simulink model "Group3_HEV_model"  (Simulink 7.9)
settings: Solver=ode4  StartTime=0.0  StopTime=Stoptime  FixedStep=1  MaxStep=.05  RelTol=1e-3
InitFcn:
  | load Mat_files/ENV_Data.mat;
  | load Mat_files/TRAN_Data.mat;
  | load Mat_files/VEH_Data.mat;
  | load Mat_files/TC_Data.mat;
  | load Mat_files/Drive_cycle.mat;
  | load Mat_files/ICE_Data.mat;
  | load Mat_files/EM_Data.mat;
  | load Mat_files/BATT_Data.mat
  | clc;
  | %warning off all;
StopFcn:
  | disp('Simulation Complete.')
values from neighbouring files (symbols this model uses):
  EM = EM2    [Group3_Plot.m]
  EM2 =     [EM2_map.mat]
  em_trq_e_g1 = em_trq_e    [Group3_ECMS_control_strategy.m]    (also in ecms_table_n5.mat = [-2 -2 -2 -2 -2 -2 -2 -2 -2 -2 -2 -2 ... (715 elements, 11x1)
  em_trq_e_g2 = em_trq_e    [Group3_ECMS_control_strategy.m]    (also in ecms_table_n5.mat = [-2 -2 -2 -2 -2 -2 -2 -2 -2 -2 -2 -2 ... (715 elements, 11x1)
  em_trq_e_g3 = em_trq_e    [Group3_ECMS_control_strategy.m]    (also in ecms_table_n5.mat = [-2 -2 -2 -2 -2 -2 -2 -2 -2 -2 -2 -2 ... (715 elements, 11x1)
  fs_0 = 1    [Group3_Initialization.m]
  fs_act = 1    [Group3_Initialization.m]
  hA_0 = 0.07    [Group3_Initialization.m]
  ICE =     [Engine2_map.mat]
  ice_w_e = linspace(0,50*m2,m2+1)    [Group3_ECMS_control_strategy.m]    (also in ecms_table_n5.mat = [0 50 100 150 200 250 300 350 400 450 500])
  mc = 50    [Group3_Initialization.m]
  N = 250    [Group3_Initialization.m]
  soc_e = linspace(-1,1,m3)    [Group3_ECMS_control_strategy.m]    (also in ecms_table_n5.mat = [-1 -0.5 0 0.5 1])
  soc_h = 0.85    [Group3_ECMS_control_strategy.m]    (also in Group3_Initialization.m)
  soc_l = 0.55    [Group3_ECMS_control_strategy.m]    (also in Group3_Initialization.m)
  Sport = 1    [Group3_Initialization.m]
  T_amb = 20+273    (= 293)    [Group3_Initialization.m]
  Treq = linspace(0,20*m1,m1+1)    [Group3_ECMS_control_strategy.m]    (also in ecms_table_n5.mat = [0 20 40 60 80 100 120 140 160 180 200 220 ... (13 elements,)
undefined symbols (not defined in the file or in its folder): BATT, ENV, TC, TRAN, VEH
libraries: simulink x6
(part 1 of 2)
settings Model: Creator=pisup  LastModifiedBy=HarryBrown
settings OptimizationCC: InitFltsAndDblsToZero=on
settings DebuggingCC: SaveWithParameterizedLinksMsg=none  CheckSSInitialOutputMsg=off  SignalResolutionControl=TryResolveAllWithWarning  MultiTaskDSMMsg=warning  MultiTaskCondExecSysMsg=none  StrictBusMsg=None
settings RTWCC: IncludeERTFirstTime=on
settings CodeAppCC: CustomSymbolStrType=$N$R$M_T
settings GRTTargetCC: TargetFcnLib=ansi_tfl_tmw.mat  CombineOutputUpdateFcns=off  GRTInterface=on

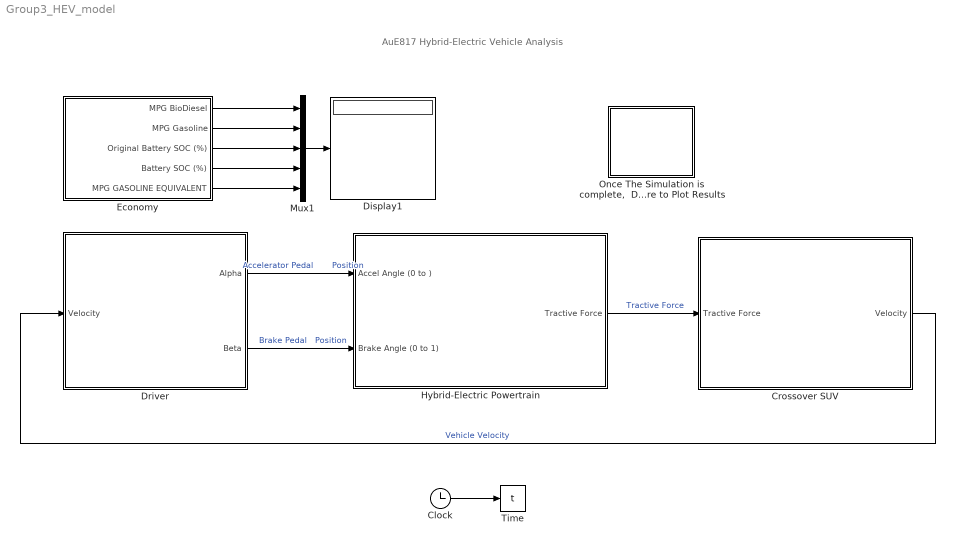
== system Group3_HEV_model ==
  note: AuE817
      | Hybrid-Electric Vehicle Analysis
  Clock : Clock
  Crossover SUV : Subsystem
      mask Type: Vehicle
      mask Display: image(imread('Images\Equinox.jpg'))
  Display1 : Display
  Driver : Subsystem
      mask Display: image(imread('Images\Driver.jpg'))
  Economy : Subsystem
      mask Type: Fuel Economy
  Hybrid-Electric Powertrain : Subsystem
      mask Display: image(imread('Images\PT.jpg'))
  Mux1 : Mux  Inputs=5
  "Once The Simulation is complete,  Double Click Here to Plot Results" : Subsystem
      settings: OpenFcn=eval 'Plot_Results'
  Time : ToWorkspace  VariableName=t  SampleTime=-1
  wires:
  Crossover SUV/1(Velocity) -> Driver/1(" Velocity")  "Vehicle Velocity"
  Driver/2(Beta) -> Hybrid-Electric Powertrain/2("Brake Angle (0 to 1) ")  "Brake Pedal   Position"
  Driver/1(Alpha) -> Hybrid-Electric Powertrain/1("Accel Angle (0 to ) ")  "Accelerator Pedal       Position"
  Hybrid-Electric Powertrain/1(Tractive Force) -> Crossover SUV/1(Tractive Force)  "Tractive Force"
  Clock/1 -> Time/1
  Mux1/1 -> Display1/1
  Economy/1(MPG BioDiesel) -> Mux1/1
  Economy/2(MPG Gasoline) -> Mux1/2
  Economy/3(Original Battery SOC (%)) -> Mux1/3
  Economy/5(MPG GASOLINE EQUIVALENT) -> Mux1/5
  Economy/4(Battery SOC (%)) -> Mux1/4

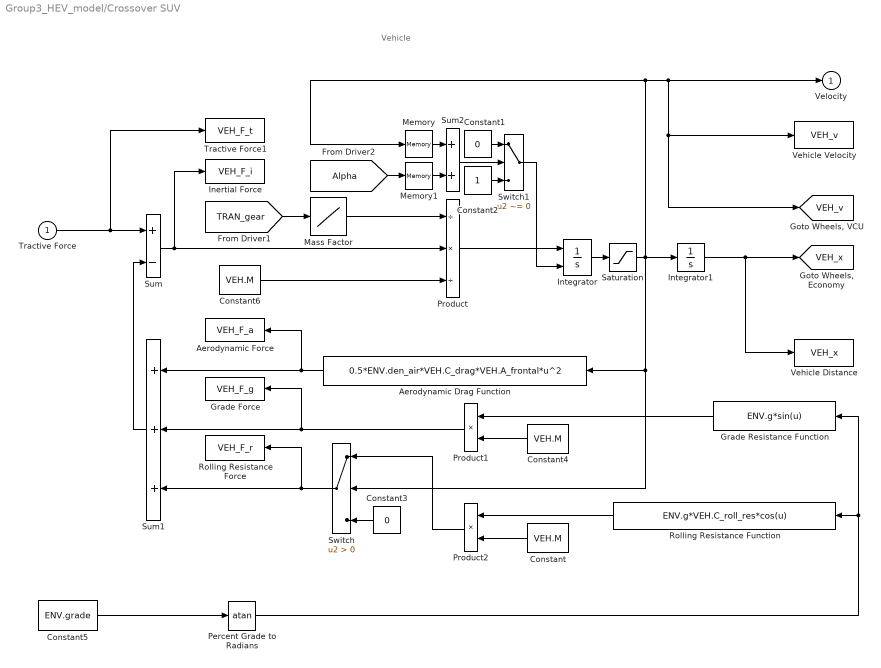
== system Group3_HEV_model/Crossover SUV ==
  note: Vehicle
  Tractive Force : Inport
  Aerodynamic Drag Function : Fcn  Expr=0.5*ENV.den_air*VEH.C_drag*VEH.A_frontal*u^2
  Aerodynamic Force : ToWorkspace  VariableName=VEH_F_a  SampleTime=-1
  Constant : Constant  Value=VEH.M
  Constant1 : Constant  Value=0
  Constant2 : Constant
  Constant3 : Constant  Value=0
  Constant4 : Constant  Value=VEH.M
  Constant5 : Constant  Value=ENV.grade
  Constant6 : Constant  Value=VEH.M
  Grade Force : ToWorkspace  VariableName=VEH_F_g  SampleTime=-1
  Grade Resistance Function : Fcn  Expr=ENV.g*sin(u)
  Inertial Force : ToWorkspace  VariableName=VEH_F_i  SampleTime=-1
  Integrator : Integrator  ExternalReset=level  LowerSaturationLimit=0
  Integrator1 : Integrator
  Mass Factor : Lookup  InputValues=[1 2 3 4 5 6]  Table=[1.7896 1.3703 1.2188 1.1536 1.1093 1.085]  SaturateOnIntegerOverflow=on
  Memory : Memory
  Memory1 : Memory
  Percent Grade to Radians : Trigonometry  Operator=atan
  Product : Product  Inputs=/*/  RndMeth=Zero
  Product1 : Product  Inputs=**  RndMeth=Zero
  Product2 : Product  Inputs=**  RndMeth=Zero
  Rolling Resistance Force : ToWorkspace  VariableName=VEH_F_r  SampleTime=-1
  Rolling Resistance Function : Fcn  Expr=ENV.g*VEH.C_roll_res*cos(u)
  Saturation : Saturate  UpperLimit=inf  LowerLimit=0
  Sum : Sum  Inputs=+-  SaturateOnIntegerOverflow=on  InputSameDT=on  OutDataTypeStr=Inherit: Same as first input
  Sum1 : Sum  Inputs=+++  SaturateOnIntegerOverflow=on  InputSameDT=on  OutDataTypeStr=Inherit: Same as first input
  Sum2 : Sum  SaturateOnIntegerOverflow=on  InputSameDT=on  OutDataTypeStr=Inherit: Same as first input
  Switch : Switch  Criteria=u2 > Threshold  SaturateOnIntegerOverflow=on  InputSameDT=on
  Switch1 : Switch  Criteria=u2 ~= 0  SaturateOnIntegerOverflow=on  InputSameDT=on
  Tractive Force1 : ToWorkspace  VariableName=VEH_F_t  SampleTime=-1
  Vehicle Distance : ToWorkspace  VariableName=VEH_x  SampleTime=-1
  Vehicle Velocity : ToWorkspace  VariableName=VEH_v  SampleTime=-1
  Velocity : Outport  InitialOutput=0
  tag scope: VEH_v=global, VEH_x=global
  wires:
  Sum1/1 -> Sum/2
  Tractive Force/1 -> Sum/1, Tractive Force1/1
  Aerodynamic Drag Function/1 -> Aerodynamic Force/1, Sum1/1
  Integrator1/1 -> [VEH_x], Vehicle Distance/1
  Constant3/1 -> Switch/3
  Sum/1 -> Inertial Force/1, Product/2
  Integrator/1 -> Saturation/1
  Switch/1 -> Sum1/3, Rolling Resistance Force/1
  Constant5/1 -> Percent Grade to Radians/1
  Percent Grade to Radians/1 -> Grade Resistance Function/1, Rolling Resistance Function/1
  Product/1 -> Integrator/1
  Mass Factor/1 -> Product/1
  [TRAN_gear] -> Mass Factor/1
  Saturation/1 -> Integrator1/1, Switch/2, Aerodynamic Drag Function/1, Vehicle Velocity/1, [VEH_v], Velocity/1, Memory/1
  [Alpha] -> Memory1/1
  Sum2/1 -> Switch1/2
  Switch1/1 -> Integrator/2
  Constant1/1 -> Switch1/1
  Constant2/1 -> Switch1/3
  Memory1/1 -> Sum2/2
  Memory/1 -> Sum2/1
  Constant6/1 -> Product/3
  Grade Resistance Function/1 -> Product1/1
  Product1/1 -> Sum1/2, Grade Force/1
  Constant4/1 -> Product1/2
  Constant/1 -> Product2/2
  Rolling Resistance Function/1 -> Product2/1
  Product2/1 -> Switch/1

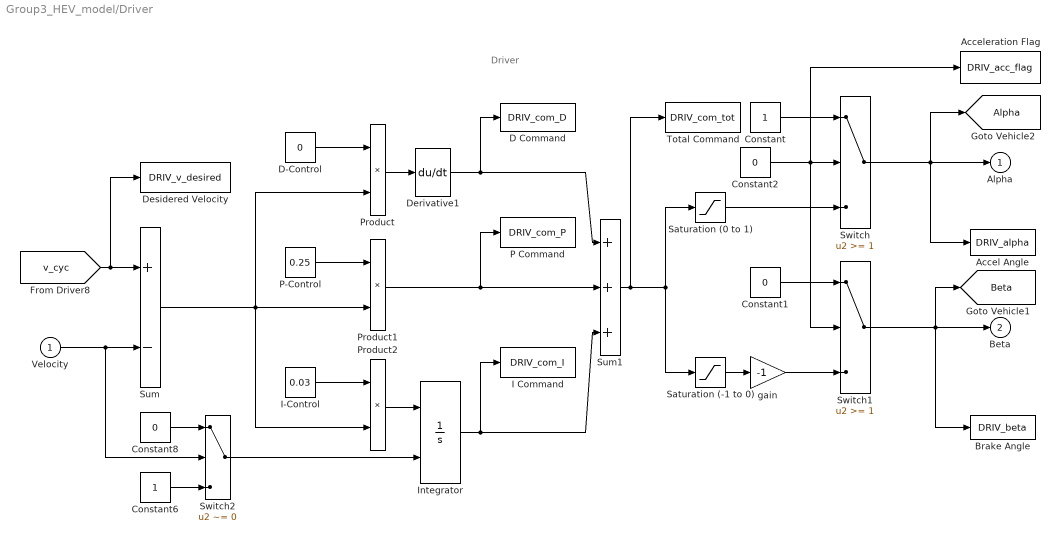
== system Group3_HEV_model/Driver ==
  note: Driver
  " Velocity" : Inport
  Accel Angle : ToWorkspace  VariableName=DRIV_alpha  SampleTime=-1
  Acceleration Flag : ToWorkspace  VariableName=DRIV_acc_flag  SampleTime=-1
  Brake Angle : ToWorkspace  VariableName=DRIV_beta  SampleTime=-1
  Constant : Constant
  Constant1 : Constant  Value=0
  Constant2 : Constant  Value=0
  Constant6 : Constant
  Constant8 : Constant  Value=0
  D Command : ToWorkspace  VariableName=DRIV_com_D  SampleTime=-1
  D-Control : Constant  Value=0
  Derivative1 : Derivative
  Desidered Velocity : ToWorkspace  VariableName=DRIV_v_desired  SampleTime=-1
  I Command : ToWorkspace  VariableName=DRIV_com_I  SampleTime=-1
  I-Control : Constant  Value=0.03
  Integrator : Integrator  ExternalReset=level
  P Command : ToWorkspace  VariableName=DRIV_com_P  SampleTime=-1
  P-Control : Constant  Value=0.25
  Product : Product  RndMeth=Zero
  Product1 : Product  RndMeth=Zero
  Product2 : Product  RndMeth=Zero
  Saturation (-1 to 0) : Saturate  UpperLimit=0  LowerLimit=-1
  Saturation (0 to 1) : Saturate  UpperLimit=1  LowerLimit=0
  Sum : Sum  Inputs=+-  SaturateOnIntegerOverflow=on  InputSameDT=on  OutDataTypeStr=Inherit: Same as first input
  Sum1 : Sum  Inputs=+++  SaturateOnIntegerOverflow=on  InputSameDT=on  OutDataTypeStr=Inherit: Same as first input
  Switch : Switch  Threshold=1  SaturateOnIntegerOverflow=on  InputSameDT=on
  Switch1 : Switch  Threshold=1  SaturateOnIntegerOverflow=on  InputSameDT=on
  Switch2 : Switch  Criteria=u2 ~= 0  Threshold=1  SaturateOnIntegerOverflow=on  InputSameDT=on
  Total Command : ToWorkspace  VariableName=DRIV_com_tot  SampleTime=-1
  gain : Gain  Gain=-1  SaturateOnIntegerOverflow=on  OutDataTypeStr=Inherit: Same as input  ParamDataTypeStr=Inherit: Same as input
  Alpha : Outport  InitialOutput=0
  Beta : Outport  Port=2  InitialOutput=0
  tag scope: Alpha=global, Beta=global
  wires:
  Switch/1 -> Accel Angle/1, Alpha/1, [Alpha]
  Constant1/1 -> Switch1/1
  gain/1 -> Switch1/3
  Saturation (0 to 1)/1 -> Switch/3
  Constant/1 -> Switch/1
  Constant2/1 -> Switch/2, Acceleration Flag/1, Switch1/2
  Saturation (-1 to 0)/1 -> gain/1
  Sum1/1 -> Saturation (-1 to 0)/1, Saturation (0 to 1)/1, Total Command/1
  " Velocity"/1 -> Sum/2, Switch2/2
  Switch1/1 -> Beta/1, Brake Angle/1, [Beta]
  Sum/1 -> Product/2, Product1/2, Product2/2
  Derivative1/1 -> Sum1/1, D Command/1
  Product/1 -> Derivative1/1
  Product1/1 -> P Command/1, Sum1/2
  Product2/1 -> Integrator/1
  Constant6/1 -> Switch2/3
  Integrator/1 -> Sum1/3, I Command/1
  Switch2/1 -> Integrator/2
  Constant8/1 -> Switch2/1
  [v_cyc] -> Sum/1, Desidered Velocity/1
  D-Control/1 -> Product/1
  P-Control/1 -> Product1/1
  I-Control/1 -> Product2/1

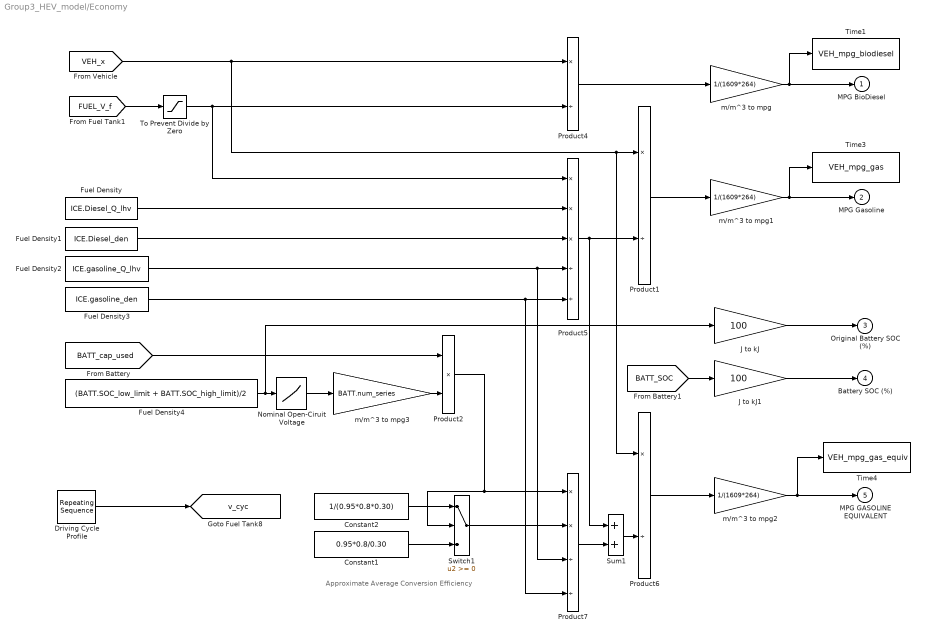
== system Group3_HEV_model/Economy ==
  note: Approximate
      | Average Conversion Efficiency
  Constant1 : Constant  Value=0.95*0.8/0.30
  Constant2 : Constant  Value=1/(0.95*0.8*0.30)
  Driving Cycle Profile : simulink/Sources/Repeating Sequence  rep_seq_t=t_cyc  rep_seq_y=v_cyc
  Fuel Density : Constant  Value=ICE.Diesel_Q_lhv
  Fuel Density1 : Constant  Value=ICE.Diesel_den
  Fuel Density2 : Constant  Value=ICE.gasoline_Q_lhv
  Fuel Density3 : Constant  Value=ICE.gasoline_den
  Fuel Density4 : Constant  Value=(BATT.SOC_low_limit + BATT.SOC_high_limit)/2
  J to kJ : Gain  Gain=100  SaturateOnIntegerOverflow=on  OutDataTypeStr=Inherit: Same as input  ParamDataTypeStr=Inherit: Same as input
  J to kJ1 : Gain  Gain=100  SaturateOnIntegerOverflow=on  OutDataTypeStr=Inherit: Same as input  ParamDataTypeStr=Inherit: Same as input
  Nominal Open-Ciruit Voltage : Lookup  InputValues=BATT.V_oc_SOC  Table=BATT.V_oc  SaturateOnIntegerOverflow=on
  Product1 : Product  Inputs=*/  SaturateOnIntegerOverflow=on  InputSameDT=on  OutDataTypeStr=Inherit: Same as first input
  Product2 : Product  Inputs=**  SaturateOnIntegerOverflow=on  InputSameDT=on  OutDataTypeStr=Inherit: Same as first input
  Product4 : Product  Inputs=*/  SaturateOnIntegerOverflow=on  InputSameDT=on  OutDataTypeStr=Inherit: Same as first input
  Product5 : Product  Inputs=***//  SaturateOnIntegerOverflow=on  InputSameDT=on  OutDataTypeStr=Inherit: Same as first input
  Product6 : Product  Inputs=*/  SaturateOnIntegerOverflow=on  InputSameDT=on  OutDataTypeStr=Inherit: Same as first input
  Product7 : Product  Inputs=**//  SaturateOnIntegerOverflow=on  InputSameDT=on  OutDataTypeStr=Inherit: Same as first input
  Sum1 : Sum  SaturateOnIntegerOverflow=on  InputSameDT=on  OutDataTypeStr=Inherit: Same as first input
  Switch1 : Switch  SaturateOnIntegerOverflow=on  InputSameDT=on
  Time1 : ToWorkspace  VariableName=VEH_mpg_biodiesel  SampleTime=-1
  Time3 : ToWorkspace  VariableName=VEH_mpg_gas  SampleTime=-1
  Time4 : ToWorkspace  VariableName=VEH_mpg_gas_equiv  SampleTime=-1
  To Prevent Divide by Zero : Saturate  UpperLimit=inf  LowerLimit=0.000001
  m/m^3 to mpg : Gain  Gain=1/(1609*264)  SaturateOnIntegerOverflow=on  OutDataTypeStr=Inherit: Same as input  ParamDataTypeStr=Inherit: Same as input
  m/m^3 to mpg1 : Gain  Gain=1/(1609*264)  SaturateOnIntegerOverflow=on  OutDataTypeStr=Inherit: Same as input  ParamDataTypeStr=Inherit: Same as input
  m/m^3 to mpg2 : Gain  Gain=1/(1609*264)  SaturateOnIntegerOverflow=on  OutDataTypeStr=Inherit: Same as input  ParamDataTypeStr=Inherit: Same as input
  m/m^3 to mpg3 : Gain  Gain=BATT.num_series  SaturateOnIntegerOverflow=on  OutDataTypeStr=Inherit: Same as input  ParamDataTypeStr=Inherit: Same as input
  MPG BioDiesel : Outport  InitialOutput=0
  MPG Gasoline : Outport  Port=2  InitialOutput=0
  Original Battery SOC (%) : Outport  Port=3  InitialOutput=0
  Battery SOC (%) : Outport  Port=4  InitialOutput=0
  MPG GASOLINE EQUIVALENT : Outport  Port=5  InitialOutput=0
  tag scope: v_cyc=global
  wires:
  [VEH_x] -> Product4/1, Product1/1, Product6/1
  m/m^3 to mpg/1 -> Time1/1, MPG BioDiesel/1
  [FUEL_V_f] -> To Prevent Divide by Zero/1
  Product4/1 -> m/m^3 to mpg/1
  Product1/1 -> m/m^3 to mpg1/1
  Fuel Density/1 -> Product5/2
  Fuel Density1/1 -> Product5/3
  Fuel Density2/1 -> Product5/4, Product7/3
  Fuel Density3/1 -> Product5/5, Product7/4
  J to kJ/1 -> Original Battery SOC (%)/1
  m/m^3 to mpg2/1 -> MPG GASOLINE EQUIVALENT/1, Time4/1
  Product6/1 -> m/m^3 to mpg2/1
  Sum1/1 -> Product6/2
  Product7/1 -> Sum1/2
  Constant2/1 -> Switch1/1
  Constant1/1 -> Switch1/3
  Switch1/1 -> Product7/2
  Product5/1 -> Sum1/1, Product1/2
  To Prevent Divide by Zero/1 -> Product4/2, Product5/1
  Fuel Density4/1 -> Nominal Open-Ciruit Voltage/1, J to kJ/1
  Nominal Open-Ciruit Voltage/1 -> m/m^3 to mpg3/1
  [BATT_cap_used] -> Product2/1
  m/m^3 to mpg3/1 -> Product2/2
  Product2/1 -> Product7/1, Switch1/2
  m/m^3 to mpg1/1 -> Time3/1, MPG Gasoline/1
  J to kJ1/1 -> Battery SOC (%)/1
  [BATT_SOC] -> J to kJ1/1
  Driving Cycle Profile/1 -> [v_cyc]

== system Group3_HEV_model/Hybrid-Electric Powertrain ==
  note: Powertrain
  "Accel Angle (0 to ) " : Inport
  "Brake Angle (0 to 1) " : Inport  Port=2
  Automatic Transaxle : Subsystem
      mask Display: image(imread('Images\Transaxle.jpg'))
  CONTROLLER : Subsystem
  EM Gearbox : Subsystem
      mask Display: image(imread('Images\Differential.jpg'))
  Electric Motor : Subsystem
      mask Type: Traction Electric Motor
      mask Display: image(imread('Images\Traction_Motor.jpg'));
  Front Brakes : Subsystem
      mask Display: image(imread('Images\Brake.jpg'))
  Front Wheels : Subsystem
      mask Display: image(imread('Images\Wheel.jpg'))
  Fuel Tank : Subsystem  mask(Fuel Tank){}
      mask Display: image(imread('Images\Fuel_Tank.jpg'))
  High-Voltage Battery & Switch Box2 : Subsystem
      mask Display: image(imread('Images\Battery.jpg'))
  Internal Combustion Engine : Subsystem
      mask Type: Internal Combustion Engine and Integrated Starter/Alternator Motor
      mask Display: image(imread('Images\Engine_ISA.jpg'));
  Rear Brakes : Subsystem
      mask Display: image(imread('Images\Brake.jpg'))
  Rear Wheels : Subsystem
      mask Display: image(imread('Images\Wheel.jpg'))
  Sum : Sum  Inputs=|++
  Torque Converter : Subsystem
      mask Type: Torque Converter
      mask Display: image(imread('Images\Torque_Converter.jpg'))
  Tractive Force : Outport  InitialOutput=0
  wires:
  Front Brakes/1(Torque Out) -> Front Wheels/1(Torque In)
  Automatic Transaxle/1(Torque Out) -> Front Brakes/1(Torque In)
  "Brake Angle (0 to 1) "/1 -> CONTROLLER/2(Beta)
  "Accel Angle (0 to ) "/1 -> CONTROLLER/1(Alpha)
  CONTROLLER/1(Engine State) -> Internal Combustion Engine/1(ICE State)
  Internal Combustion Engine/1(Torque Out) -> Torque Converter/2(Torque In (Pump Torque))
  Torque Converter/1(Torque Out (Turbine Torque)) -> Automatic Transaxle/2(Torque In)
  CONTROLLER/4(TC Lock-Up?) -> Torque Converter/1(Torque Converter Lock-Up?)
  CONTROLLER/5(Gear Request) -> Automatic Transaxle/1(Gear Command)
  Front Wheels/1(Tractive Force) -> Sum/1
  Rear Wheels/1(Tractive Force) -> Sum/2
  Sum/1 -> Tractive Force/1
  Rear Brakes/1(Torque Out) -> Rear Wheels/1(Torque In)
  EM Gearbox/1(Torque Out) -> Rear Brakes/1(Torque In)
  Electric Motor/1(Torque Out) -> EM Gearbox/1(Torque In)
  CONTROLLER/2(Engine Torque Request) -> Internal Combustion Engine/2(ICE Torque In (Commanded ICE Torque))
  CONTROLLER/3(Electric Motor Torque Request) -> Electric Motor/1(EM Torque In (Commanded EM Torque))

== system Group3_HEV_model/Once The Simulation is complete,  Double Click Here to Plot Results ==
  Constant : Constant
  Terminator : Terminator
  wires:
  Constant/1 -> Terminator/1

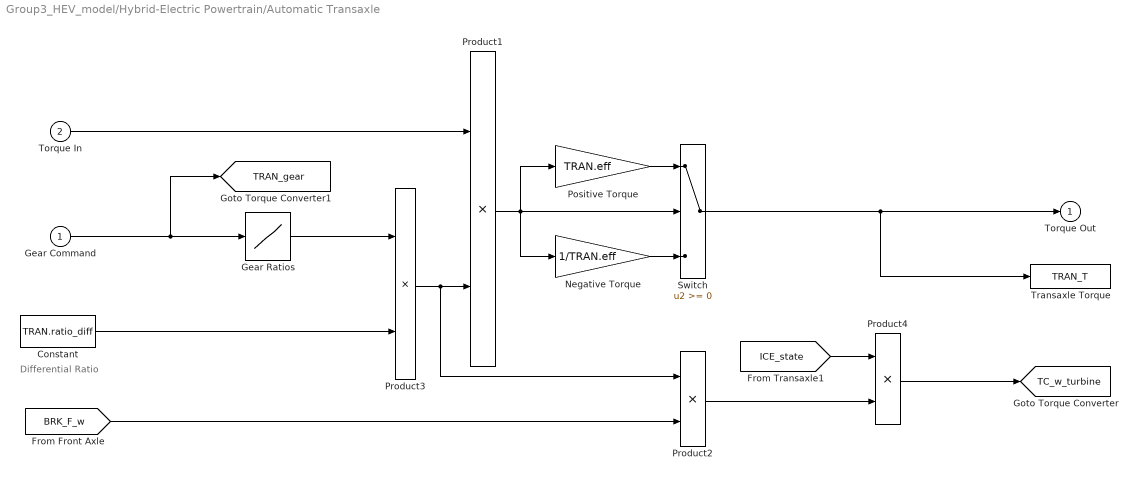
== system Group3_HEV_model/Hybrid-Electric Powertrain/Automatic Transaxle ==
  note: Differential Ratio
  Gear Command : Inport
  Torque In : Inport  Port=2
  Constant : Constant  Value=TRAN.ratio_diff
  Gear Ratios : Lookup  InputValues=[1 2 3 4]  Table=[TRAN.ratio_gear(1) TRAN.ratio_gear(2) TRAN.ratio_gear(3) TRAN.ratio_gear(4)]  SaturateOnIntegerOverflow=on
  Negative Torque : Gain  Gain=1/TRAN.eff  SaturateOnIntegerOverflow=on  OutDataTypeStr=Inherit: Same as input  ParamDataTypeStr=Inherit: Same as input
  Positive Torque : Gain  Gain=TRAN.eff  SaturateOnIntegerOverflow=on  OutDataTypeStr=Inherit: Same as input  ParamDataTypeStr=Inherit: Same as input
  Product1 : Product  SaturateOnIntegerOverflow=on  InputSameDT=on  OutDataTypeStr=Inherit: Same as first input
  Product2 : Product  SaturateOnIntegerOverflow=on  InputSameDT=on  OutDataTypeStr=Inherit: Same as first input
  Product3 : Product  SaturateOnIntegerOverflow=on  InputSameDT=on  OutDataTypeStr=Inherit: Same as first input
  Product4 : Product  Inputs=**  SaturateOnIntegerOverflow=on  InputSameDT=on  OutDataTypeStr=Inherit: Same as first input
  Switch : Switch  SaturateOnIntegerOverflow=on  InputSameDT=on
  Transaxle Torque : ToWorkspace  VariableName=TRAN_T  SampleTime=-1
  Torque Out : Outport  InitialOutput=0
  tag scope: TC_w_turbine=global, TRAN_gear=global
  wires:
  Torque In/1 -> Product1/1
  Positive Torque/1 -> Switch/1
  Product1/1 -> Switch/2, Positive Torque/1, Negative Torque/1
  Negative Torque/1 -> Switch/3
  Constant/1 -> Product3/2
  Product3/1 -> Product1/2, Product2/1
  [BRK_F_w] -> Product2/2
  Gear Command/1 -> [TRAN_gear], Gear Ratios/1
  Switch/1 -> Torque Out/1, Transaxle Torque/1
  [ICE_state] -> Product4/1
  Product2/1 -> Product4/2
  Product4/1 -> [TC_w_turbine]
  Gear Ratios/1 -> Product3/1

== system Group3_HEV_model/Hybrid-Electric Powertrain/CONTROLLER ==
  Alpha : Inport
  Beta : Inport  Port=2
  Primary Control : Subsystem
  Engine State : Outport  InitialOutput=0
  Engine Torque Request : Outport  Port=2  InitialOutput=0
  Electric Motor Torque Request : Outport  Port=3  InitialOutput=0
  TC Lock-Up? : Outport  Port=4  InitialOutput=0
  Gear Request : Outport  Port=5  InitialOutput=0
  wires:
  Alpha/1 -> Primary Control/1(Alpha)
  Beta/1 -> Primary Control/2(Beta)
  Primary Control/5(Transmission Gear) -> Gear Request/1
  Primary Control/1(Engine State) -> Engine State/1
  Primary Control/4(TC Lock-Up?) -> TC Lock-Up?/1
  Primary Control/2(Engine Torque) -> Engine Torque Request/1
  Primary Control/3(Electric Motor Torque) -> Electric Motor Torque Request/1

== system Group3_HEV_model/Hybrid-Electric Powertrain/EM Gearbox ==
  Torque In : Inport
  Differential Ratio : Constant  Value=EM.gearbox_ratio
  Divide : Product  Inputs=**
  Divide1 : Product
  Negative Torque : Gain  Gain=1/EM.gearbox_eff  SaturateOnIntegerOverflow=on  OutDataTypeStr=Inherit: Same as input  ParamDataTypeStr=Inherit: Same as input
  Positive Torque : Gain  Gain=EM.gearbox_eff  SaturateOnIntegerOverflow=on  OutDataTypeStr=Inherit: Same as input  ParamDataTypeStr=Inherit: Same as input
  Switch : Switch  SaturateOnIntegerOverflow=on  InputSameDT=on
  Torque Out : Outport  InitialOutput=0
  tag scope: DIFF_R_w=global
  wires:
  Differential Ratio/1 -> Divide/2, Divide1/1
  Torque In/1 -> Divide/1
  [BRK_R_w] -> Divide1/2
  Positive Torque/1 -> Switch/1
  Divide/1 -> Switch/2, Positive Torque/1, Negative Torque/1
  Negative Torque/1 -> Switch/3
  Switch/1 -> Torque Out/1
  Divide1/1 -> [DIFF_R_w]

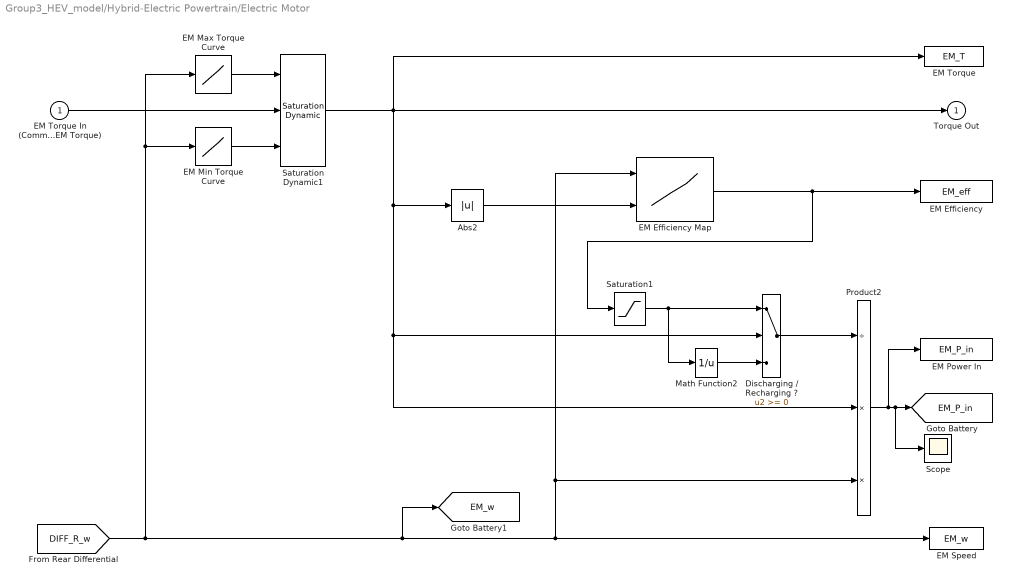
== system Group3_HEV_model/Hybrid-Electric Powertrain/Electric Motor ==
  EM Torque In (Commanded EM Torque) : Inport
  Abs2 : Abs  SaturateOnIntegerOverflow=on
  Discharging / Recharging ? : Switch  SaturateOnIntegerOverflow=on  InputSameDT=on
  EM Efficiency : ToWorkspace  VariableName=EM_eff  SampleTime=-1
  EM Efficiency Map : Lookup2D  RowIndex=EM2.map_w  ColumnIndex=EM2.map_T  Table=EM2.map_eff  SaturateOnIntegerOverflow=on
  EM Max Torque Curve : Lookup  InputValues=EM2.maxT_w  Table=EM2.maxT_T  SaturateOnIntegerOverflow=on
  EM Min Torque Curve : Lookup  InputValues=EM2.maxT_w  Table=EM2.minT_T  SaturateOnIntegerOverflow=on
  EM Power In : ToWorkspace  VariableName=EM_P_in  SampleTime=-1
  EM Speed : ToWorkspace  VariableName=EM_w  SampleTime=-1
  EM Torque : ToWorkspace  VariableName=EM_T  SampleTime=-1
  Math Function2 : Math  Operator=reciprocal  SaturateOnIntegerOverflow=on
  Product2 : Product  Inputs=/**  SaturateOnIntegerOverflow=on  InputSameDT=on  OutDataTypeStr=Inherit: Same as first input
  Saturation Dynamic1 : simulink/Discontinuities/Saturation Dynamic  OutMin=[]  OutMax=[]  OutDataTypeStr=Inherit: Same as second input  OutDataType=sfix(16)  OutScaling=2^-10  DoSatur=off
  Saturation1 : Saturate  UpperLimit=1  LowerLimit=0.001
  Scope : Scope
      settings: SaveName=ScopeData3
  Torque Out : Outport  InitialOutput=0
  tag scope: EM_P_in=global, EM_w=global
  wires:
  EM Torque In (Commanded EM Torque)/1 -> Saturation Dynamic1/2
  EM Min Torque Curve/1 -> Saturation Dynamic1/3
  EM Max Torque Curve/1 -> Saturation Dynamic1/1
  Product2/1 -> EM Power In/1, Scope/1, [EM_P_in]
  Discharging / Recharging ?/1 -> Product2/1
  EM Efficiency Map/1 -> EM Efficiency/1, Saturation1/1
  Abs2/1 -> EM Efficiency Map/2
  Saturation Dynamic1/1 -> Product2/2, Discharging / Recharging ?/2, Abs2/1, EM Torque/1, Torque Out/1
  Saturation1/1 -> Discharging / Recharging ?/1, Math Function2/1
  Math Function2/1 -> Discharging / Recharging ?/3
  [DIFF_R_w] -> EM Max Torque Curve/1, EM Min Torque Curve/1, Product2/3, EM Efficiency Map/1, EM Speed/1, [EM_w]

== system Group3_HEV_model/Hybrid-Electric Powertrain/Front Brakes ==
  Torque In : Inport
  Constant1 : Constant  Value=ENV.C_fric_tire_gnd
  Constant2 : Constant  Value=ENV.g
  Constant3 : Constant  Value=VEH.r_tire
  Constant4 : Constant  Value=VEH.M
  Gain : Gain  Gain=VEH.brake_F_propor
  Product : Product  Inputs=5  RndMeth=Zero
  Sum : Sum  Inputs=-+  SaturateOnIntegerOverflow=on  InputSameDT=on  OutDataTypeStr=Inherit: Same as first input
  Torque Out : Outport  InitialOutput=0
  tag scope: BRK_F_w=global
  wires:
  Product/1 -> Gain/1
  Torque In/1 -> Sum/2
  [WH_F_w] -> [BRK_F_w]
  Constant4/1 -> Product/2
  Constant1/1 -> Product/3
  Constant2/1 -> Product/4
  Constant3/1 -> Product/5
  [Beta] -> Product/1
  Gain/1 -> Sum/1
  Sum/1 -> Torque Out/1

== system Group3_HEV_model/Hybrid-Electric Powertrain/Front Wheels ==
  Torque In : Inport
  Divide : Product  Inputs=*/
  Divide1 : Product  Inputs=/*
  Front Wheel Speed : ToWorkspace  VariableName=WH_F_w  SampleTime=-1
  Front Wheel Torque : ToWorkspace  VariableName=WH_F_T  SampleTime=-1
  Wheel Radius : Constant  Value=VEH.r_tire
  Tractive Force : Outport  InitialOutput=0
  tag scope: WH_F_w=global
  wires:
  Wheel Radius/1 -> Divide/2, Divide1/1
  Torque In/1 -> Divide/1, Front Wheel Torque/1
  Divide/1 -> Tractive Force/1
  [VEH_v] -> Divide1/2
  Divide1/1 -> [WH_F_w], Front Wheel Speed/1

== system Group3_HEV_model/Hybrid-Electric Powertrain/Fuel Tank ==
  Divide1 : Product  Inputs=/*
  Fuel Density1 : Constant  Value=ICE.gasoline_den
  Fuel_left : Display
  Fuel_tank_weight : Display
  Integrator1 : Integrator
  Original_Mass_Gasoline_kg : Constant  Value=30
  Subtract2 : Sum  Inputs=-+
  Subtract3 : Sum
  Tank_mass_coefficient : Gain  Gain=0.1
  Tank_volume : Display
  Tank_volume_coefficient : Gain  Gain=1/ICE.gasoline_den*1000
  Torque Converter Torque (Nm)3 : ToWorkspace  VariableName=ICE_m_f1  SampleTime=-1
  Torque Converter Torque (Nm)4 : ToWorkspace  VariableName=FUEL_V_f1  SampleTime=-1
  tag scope: FUEL_V_f=global
  wires:
  Integrator1/1 -> Divide1/2, Torque Converter Torque (Nm)3/1, Subtract2/1
  Fuel Density1/1 -> Divide1/1
  [ICE_m_f_dot] -> Integrator1/1
  Divide1/1 -> Torque Converter Torque (Nm)4/1, [FUEL_V_f]
  Original_Mass_Gasoline_kg/1 -> Subtract2/2, Tank_volume_coefficient/1, Tank_mass_coefficient/1
  Subtract2/1 -> Subtract3/1, Fuel_left/1
  Tank_mass_coefficient/1 -> Subtract3/2
  Tank_volume_coefficient/1 -> Tank_volume/1
  Subtract3/1 -> Fuel_tank_weight/1

== system Group3_HEV_model/Hybrid-Electric Powertrain/High-Voltage Battery & Switch Box2 ==
  Battery State-of-Charge : ToWorkspace  VariableName=BATT_SOC  SampleTime=-1
  Battery State-of-Charge1 : ToWorkspace  VariableName=BATT_i  SampleTime=-1
  Battery State-of-Charge2 : ToWorkspace  VariableName=BATT_V_oc  SampleTime=-1
  Battery volume & weight : Display
  Capacity : Constant  Value=BATT.Ah
  Cell number : Constant  Value=BATT.num_series
  Mux : Mux  Inputs=2
  Nominal voltage : Constant  Value=BATT.V0
  Product : Product  Inputs=3  RndMeth=Zero
  R Circuit : Subsystem
  Subsystem : Subsystem
  volume_liter : Gain  Gain=1/40
  weight_kg : Gain  Gain=1.8/60
  tag scope: BATT_SOC=global
  wires:
  R Circuit/1(Current) -> Battery State-of-Charge1/1, Subsystem/1(Current)
  R Circuit/2(Open Circuit Voltage) -> Battery State-of-Charge2/1
  [EM_P_in] -> R Circuit/2(Power from Battery)
  Subsystem/1(Battery SOC) -> [BATT_SOC], R Circuit/1(SOC), Battery State-of-Charge/1
  Cell number/1 -> Product/1
  Capacity/1 -> Product/2
  Nominal voltage/1 -> Product/3
  Product/1 -> weight_kg/1, volume_liter/1
  Mux/1 -> Battery volume & weight/1
  weight_kg/1 -> Mux/1
  volume_liter/1 -> Mux/2

== system Group3_HEV_model/Hybrid-Electric Powertrain/Internal Combustion Engine ==
  ICE State : Inport
  ICE Torque In (Commanded ICE Torque) : Inport  Port=2
  Constant3 : Constant  Value=0
  ICE Fuel Rate In (kg/s) : ToWorkspace  VariableName=ICE_m_f_dot  SampleTime=-1
  ICE Mass Flow Rate Map (kg/s) : Lookup2D  RowIndex=ICE.map_w  ColumnIndex=ICE.map_T  Table=ICE.map_m_dot  SaturateOnIntegerOverflow=on  InputSameDT=on
  ICE Max Torque Curve : Lookup  InputValues=ICE.maxT_w  Table=ICE.maxT_T  SaturateOnIntegerOverflow=on
  ICE Speed : ToWorkspace  VariableName=ICE_w  SampleTime=-1
  ICE Torque (Nm) : ToWorkspace  VariableName=ICE_T  SampleTime=-1
  Product3 : Product  Inputs=**  SaturateOnIntegerOverflow=on  InputSameDT=on  OutDataTypeStr=Inherit: Same as first input
  Saturation Dynamic : simulink/Discontinuities/Saturation Dynamic  OutMin=[]  OutMax=[]  OutDataTypeStr=Inherit: Same as second input  OutDataType=sfix(16)  OutScaling=2^-10  DoSatur=off
  Zero Flow Rate Minimum : Saturate  UpperLimit=inf  LowerLimit=0
  Torque Out : Outport  InitialOutput=0
  tag scope: ICE_m_f_dot=global, ICE_state=global, ICE_w=global
  wires:
  ICE Max Torque Curve/1 -> Saturation Dynamic/1
  ICE Mass Flow Rate Map (kg/s)/1 -> Zero Flow Rate Minimum/1
  Product3/1 -> ICE Fuel Rate In (kg/s)/1, [ICE_m_f_dot]
  ICE State/1 -> [ICE_state], Product3/1
  ICE Torque In (Commanded ICE Torque)/1 -> Saturation Dynamic/2
  Saturation Dynamic/1 -> ICE Mass Flow Rate Map (kg/s)/2, ICE Torque (Nm)/1, Torque Out/1
  Constant3/1 -> Saturation Dynamic/3
  [TC_w_pump] -> ICE Mass Flow Rate Map (kg/s)/1, ICE Max Torque Curve/1, [ICE_w], ICE Speed/1
  Zero Flow Rate Minimum/1 -> Product3/2

== system Group3_HEV_model/Hybrid-Electric Powertrain/Rear Brakes ==
  Torque In : Inport
  Constant1 : Constant  Value=ENV.C_fric_tire_gnd
  Constant2 : Constant  Value=ENV.g
  Constant3 : Constant  Value=VEH.r_tire
  Constant4 : Constant  Value=VEH.M
  Gain : Gain  Gain=VEH.brake_R_propor
  Product : Product  Inputs=5  RndMeth=Zero
  Sum : Sum  Inputs=-+  SaturateOnIntegerOverflow=on  InputSameDT=on  OutDataTypeStr=Inherit: Same as first input
  Torque Out : Outport  InitialOutput=0
  tag scope: BRK_R_w=global
  wires:
  Sum/1 -> Torque Out/1
  Product/1 -> Gain/1
  Torque In/1 -> Sum/2
  [WH_R_w] -> [BRK_R_w]
  Constant4/1 -> Product/2
  Constant1/1 -> Product/3
  Constant2/1 -> Product/4
  Constant3/1 -> Product/5
  [Beta] -> Product/1
  Gain/1 -> Sum/1

== system Group3_HEV_model/Hybrid-Electric Powertrain/Rear Wheels ==
  Torque In : Inport
  Divide : Product  Inputs=*/
  Divide1 : Product  Inputs=/*
  Rear Wheel Speed : ToWorkspace  VariableName=WH_R_w  SampleTime=-1
  Rear Wheel Torque : ToWorkspace  VariableName=WH_R_T  SampleTime=-1
  Scope : Scope
      settings: SaveName=ScopeData11
  Wheel Radius : Constant  Value=VEH.r_tire
  Tractive Force : Outport  InitialOutput=0
  tag scope: WH_R_w=global
  wires:
  Wheel Radius/1 -> Divide/2, Divide1/1
  Torque In/1 -> Divide/1, Rear Wheel Torque/1
  Divide/1 -> Tractive Force/1
  [VEH_v] -> Scope/1, Divide1/2
  Divide1/1 -> [WH_R_w], Rear Wheel Speed/1

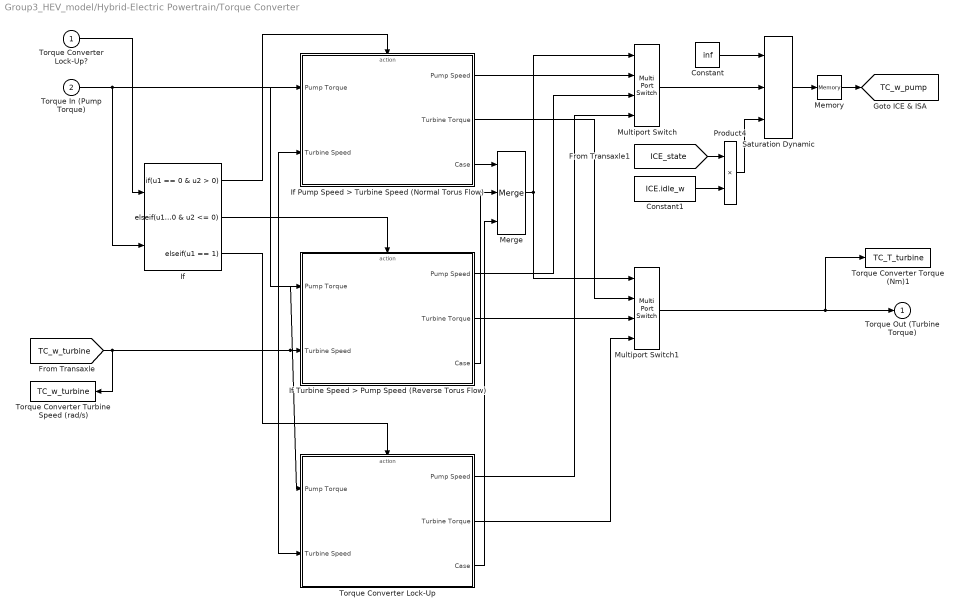
== system Group3_HEV_model/Hybrid-Electric Powertrain/Torque Converter ==
  Torque Converter Lock-Up? : Inport
  Torque In (Pump Torque) : Inport  Port=2
  Constant : Constant  Value=inf
  Constant1 : Constant  Value=ICE.idle_w
  If : If  NumInputs=2  IfExpression=u1 == 0 & u2 > 0  ElseIfExpressions=u1 == 0 & u2 <= 0, u1 == 1  ShowElse=off
  If Pump Speed > Turbine Speed (Normal Torus Flow) : Subsystem  TreatAsAtomicUnit=on
  If Turbine Speed > Pump Speed (Reverse Torus Flow) : Subsystem  TreatAsAtomicUnit=on
  Memory : Memory
  Merge : Merge  Inputs=3
  Multiport Switch : MultiPortSwitch  zeroidx=off
  Multiport Switch1 : MultiPortSwitch  zeroidx=off
  Product4 : Product  Inputs=**  SaturateOnIntegerOverflow=on  InputSameDT=on  OutDataTypeStr=Inherit: Same as first input
  Saturation Dynamic : simulink/Discontinuities/Saturation Dynamic  OutMin=[]  OutMax=[]  OutDataTypeStr=Inherit: Same as second input  OutDataType=sfix(16)  OutScaling=2^-10  DoSatur=off
  Torque Converter Turbine Speed (rad/s) : ToWorkspace  VariableName=TC_w_turbine  SampleTime=-1
  Torque Converter Lock-Up : Subsystem  TreatAsAtomicUnit=on
  Torque Converter Torque (Nm)1 : ToWorkspace  VariableName=TC_T_turbine  SampleTime=-1
  Torque Out (Turbine Torque) : Outport  InitialOutput=0
  tag scope: TC_w_pump=global
  wires:
  [TC_w_turbine] -> If Turbine Speed > Pump Speed (Reverse Torus Flow)/2(Turbine Speed), If Pump Speed > Turbine Speed (Normal Torus Flow)/2(Turbine Speed), Torque Converter Lock-Up/2(Turbine Speed), Torque Converter Turbine Speed (rad/s)/1
  If Pump Speed > Turbine Speed (Normal Torus Flow)/1(Pump Speed) -> Multiport Switch/2
  If Turbine Speed > Pump Speed (Reverse Torus Flow)/1(Pump Speed) -> Multiport Switch/3
  Multiport Switch1/1 -> Torque Out (Turbine Torque)/1, Torque Converter Torque (Nm)1/1
  Torque In (Pump Torque)/1 -> If Pump Speed > Turbine Speed (Normal Torus Flow)/1(Pump Torque), If Turbine Speed > Pump Speed (Reverse Torus Flow)/1(Pump Torque), Torque Converter Lock-Up/1(Pump Torque), If/2
  Memory/1 -> [TC_w_pump]
  If/2 -> If Turbine Speed > Pump Speed (Reverse Torus Flow)/Action
  If/1 -> If Pump Speed > Turbine Speed (Normal Torus Flow)/Action
  If/3 -> Torque Converter Lock-Up/Action
  Torque Converter Lock-Up?/1 -> If/1
  Torque Converter Lock-Up/3(Case) -> Merge/3
  Torque Converter Lock-Up/1(Pump Speed) -> Multiport Switch/4
  Merge/1 -> Multiport Switch/1, Multiport Switch1/1
  If Pump Speed > Turbine Speed (Normal Torus Flow)/3(Case) -> Merge/1
  If Turbine Speed > Pump Speed (Reverse Torus Flow)/3(Case) -> Merge/2
  If Turbine Speed > Pump Speed (Reverse Torus Flow)/2(Turbine Torque) -> Multiport Switch1/3
  Torque Converter Lock-Up/2(Turbine Torque) -> Multiport Switch1/4
  If Pump Speed > Turbine Speed (Normal Torus Flow)/2(Turbine Torque) -> Multiport Switch1/2
  Saturation Dynamic/1 -> Memory/1
  Constant/1 -> Saturation Dynamic/1
  [ICE_state] -> Product4/1
  Constant1/1 -> Product4/2
  Product4/1 -> Saturation Dynamic/3
  Multiport Switch/1 -> Saturation Dynamic/2

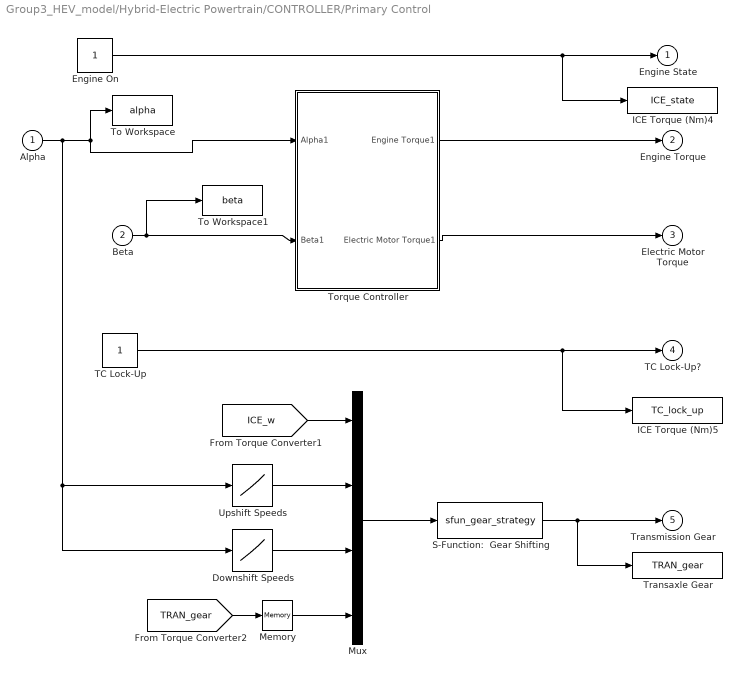
== system Group3_HEV_model/Hybrid-Electric Powertrain/CONTROLLER/Primary Control ==
  Alpha : Inport
  Beta : Inport  Port=2
  Downshift Speeds : Lookup  InputValues=[0 0.333 0.667 1]  Table=[85 85 85 85]  SaturateOnIntegerOverflow=on
  Engine On : Constant
  ICE Torque (Nm)4 : ToWorkspace  VariableName=ICE_state  SampleTime=-1
  ICE Torque (Nm)5 : ToWorkspace  VariableName=TC_lock_up  SampleTime=-1
  Memory : Memory  X0=1
  Mux : Mux
  S-Function:  Gear Shifting : S-Function  FunctionName=sfun_gear_strategy  EnableBusSupport=off
  TC Lock-Up : Constant
  To Workspace : ToWorkspace  VariableName=alpha  SampleTime=-1  SaveFormat=Timeseries
  To Workspace1 : ToWorkspace  VariableName=beta  SampleTime=-1  SaveFormat=Timeseries
  Torque Controller : Subsystem
  Transaxle Gear : ToWorkspace  VariableName=TRAN_gear  SampleTime=-1
  Upshift Speeds : Lookup  InputValues=[0, 0.333 0.667, 1]  Table=[157 209 262 660 ]  SaturateOnIntegerOverflow=on
  Engine State : Outport  InitialOutput=0
  Engine Torque : Outport  Port=2  InitialOutput=0
  Electric Motor Torque : Outport  Port=3  InitialOutput=0
  TC Lock-Up? : Outport  Port=4  InitialOutput=0
  Transmission Gear : Outport  Port=5  InitialOutput=0
  wires:
  Engine On/1 -> Engine State/1, ICE Torque (Nm)4/1
  S-Function:  Gear Shifting/1 -> Transmission Gear/1, Transaxle Gear/1
  Alpha/1 -> Downshift Speeds/1, Upshift Speeds/1, To Workspace/1, Torque Controller/1(Alpha1)
  TC Lock-Up/1 -> ICE Torque (Nm)5/1, TC Lock-Up?/1
  Downshift Speeds/1 -> Mux/3
  Upshift Speeds/1 -> Mux/2
  [ICE_w] -> Mux/1
  [TRAN_gear] -> Memory/1
  Mux/1 -> S-Function:  Gear Shifting/1
  Memory/1 -> Mux/4
  Torque Controller/1(Engine Torque1) -> Engine Torque/1
  Beta/1 -> To Workspace1/1, Torque Controller/2(Beta1)
  Torque Controller/2(Electric Motor Torque1) -> Electric Motor Torque/1

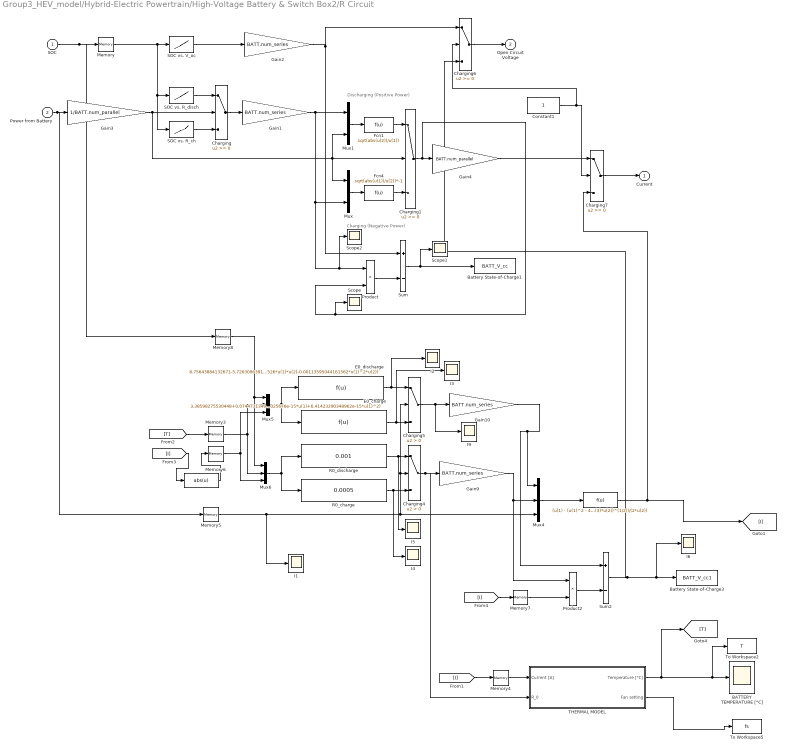
== system Group3_HEV_model/Hybrid-Electric Powertrain/High-Voltage Battery & Switch Box2/R Circuit ==
  note: Charging (Negative Power)
  note: Discharging (Positive Power)
  SOC : Inport
  Power from Battery : Inport  Port=2
  " " : Fcn  Expr=abs(u)
  "   " : Fcn  Expr=(u(1) - (u(1)^2 - 4*u(3)*u(2))^(1/2))/(2*u(2))
  BATTERY TEMPERATURE [°C] : Scope
      settings: SaveName=ScopeData13
  Battery State-of-Charge1 : ToWorkspace  VariableName=BATT_V_cc  SampleTime=-1
  Battery State-of-Charge3 : ToWorkspace  VariableName=BATT_V_cc1  SampleTime=-1
  Charging{,1,6..7} (4 alike) : Switch  SaturateOnIntegerOverflow=on  InputSameDT=on
  Charging4 : Switch  Criteria=u2 > Threshold  SaturateOnIntegerOverflow=on  InputSameDT=on
  Charging5 : Switch  Criteria=u2 > Threshold  SaturateOnIntegerOverflow=on  InputSameDT=on
  Constant1 : Constant
  E0_charge : Fcn  Expr=3.38598275530448+0.0744731349441681*u(1)-0.228280695420385*u(1)^2-u(3)*(1.00000000008258e-05-4.70154610025676e-15*u(1)+6.41423290348962e-15*u(1)^2)
  E0_discharge : Fcn  Expr=8.75643884132671-5.72630963913994*u(1)+3.89671587268422*u(1)^2-0.0187924289880750*u(2)+0.0198778941721078*u(1)*u(2)-0.0132279676497197*u(1)^2*u(2)-u(3)*(0.190881443247081-0.485824051113570*u(1)+0.365889637244396*u(1)^2-0.000561569212192113*u(2)+0.00150830192832526*u(1)*u(2)-0.00113595044161562*u(1)^2*u(2))
  Fcn1 : Fcn  Expr=sqrt(abs(u(2))/u(1))
  Fcn4 : Fcn  Expr=sqrt(abs(u(1))/u(2))*-1
  Gain{1..2,9..10} (4 alike) : Gain  Gain=BATT.num_series  SaturateOnIntegerOverflow=on  OutDataTypeStr=Inherit: Same as input  ParamDataTypeStr=Inherit: Same as input
  Gain3 : Gain  Gain=1/BATT.num_parallel  SaturateOnIntegerOverflow=on  OutDataTypeStr=Inherit: Same as input  ParamDataTypeStr=Inherit: Same as input
  Gain4 : Gain  Gain=BATT.num_parallel  SaturateOnIntegerOverflow=on  OutDataTypeStr=Inherit: Same as input  ParamDataTypeStr=Inherit: Same as input
  I{1..6,9} (7 alike) : Scope
      I1 settings: SaveName=ScopeData19
      I2 settings: SaveName=ScopeData14
      I3 settings: SaveName=ScopeData16
      I4 settings: SaveName=ScopeData17
      I5 settings: TimeRange=1360  SaveName=ScopeData18
      I6 settings: SaveName=ScopeData12
      I9 settings: SaveName=ScopeData15
  Memory{,3..8} (7 alike) : Memory
  Mux : Mux  Inputs=2
  Mux1 : Mux  Inputs=2
  Mux4 : Mux  Inputs=3
  Mux5 : Mux  Inputs=3
  Mux6 : Mux  Inputs=3
  Product : Product  RndMeth=Zero
  Product2 : Product  RndMeth=Zero
  R0_charge : Fcn  Expr=0.0005
  R0_discharge : Fcn  Expr=0.001
  SOC vs. R_ch : Lookup  InputValues=BATT.R_disch_SOC  Table=BATT.R_disch  SaturateOnIntegerOverflow=on
  SOC vs. R_disch : Lookup  InputValues=BATT.R_ch_SOC  Table=BATT.R_ch  SaturateOnIntegerOverflow=on
  SOC vs. V_oc : Lookup  InputValues=BATT.V_oc_SOC  Table=BATT.V_oc  SaturateOnIntegerOverflow=on
  Scope : Scope
      settings: SaveName=ScopeData4
  Scope1 : Scope
      settings: SaveName=ScopeData5
  Scope2 : Scope
      settings: SaveName=ScopeData6
  Sum : Sum  Inputs=+-
  Sum2 : Sum  Inputs=+-
  THERMAL MODEL : Subsystem
  To Workspace2 : ToWorkspace  VariableName=T  SampleTime=1
  To Workspace5 : ToWorkspace  VariableName=fs  SampleTime=1
  Current : Outport  InitialOutput=0
  Open Circuit Voltage : Outport  Port=2  InitialOutput=0
  wires:
  SOC vs. V_oc/1 -> Gain2/1
  Power from Battery/1 -> Gain3/1, Memory5/1
  SOC vs. R_disch/1 -> Charging/1
  SOC vs. R_ch/1 -> Charging/3
  Gain2/1 -> Sum/1, Charging6/1
  Charging/1 -> Gain1/1
  Mux/1 -> Fcn4/1
  Mux1/1 -> Fcn1/1
  Gain1/1 -> Mux1/1, Scope2/1, Product/1, Mux/2
  Sum/1 -> Scope1/1, Battery State-of-Charge1/1
  Product/1 -> Sum/2
  Gain3/1 -> Charging/2, Charging1/2, Mux1/2, Mux/1
  Fcn1/1 -> Charging1/1
  Fcn4/1 -> Charging1/3
  Charging1/1 -> Scope/1, Product/2, Gain4/1
  SOC/1 -> Memory/1, Memory8/1
  Memory/1 -> SOC vs. V_oc/1, SOC vs. R_disch/1, SOC vs. R_ch/1
  Mux4/1 -> "   "/1
  Gain9/1 -> Mux4/2, Product2/1
  Sum2/1 -> Battery State-of-Charge3/1, I6/1, Charging6/3
  Product2/1 -> Sum2/2
  THERMAL MODEL/1(Temperature [°C]) -> BATTERY TEMPERATURE [°C]/1, To Workspace2/1, [T]
  THERMAL MODEL/2(Fan setting) -> To Workspace5/1
  Mux6/1 -> R0_charge/1, R0_discharge/1
  R0_discharge/1 -> Charging4/1, I5/1
  R0_charge/1 -> Charging4/3, I4/1
  Mux5/1 -> E0_discharge/1, E0_charge/1
  E0_discharge/1 -> Charging5/1, I2/1
  E0_charge/1 -> Charging5/3, I3/1
  Charging4/1 -> Gain9/1, THERMAL MODEL/2(R_0)
  [T] -> Memory3/1
  Charging5/1 -> Gain10/1, I9/1
  Gain10/1 -> Sum2/1, Mux4/1
  [I] -> Memory4/1
  Memory4/1 -> THERMAL MODEL/1(Current [A])
  Memory5/1 -> Charging4/2, Charging5/2, Mux4/3, I1/1
  Memory6/1 -> Mux6/3, Mux5/3
  Memory3/1 -> Mux5/2, Mux6/2
  "   "/1 -> [I], Charging7/3
  [I] -> Memory7/1
  Memory7/1 -> Product2/2
  " "/1 -> Memory6/1
  [I] -> " "/1
  Constant1/1 -> Charging7/2, Charging6/2
  Charging6/1 -> Open Circuit Voltage/1
  Charging7/1 -> Current/1
  Gain4/1 -> Charging7/1
  Memory8/1 -> Mux6/1, Mux5/1

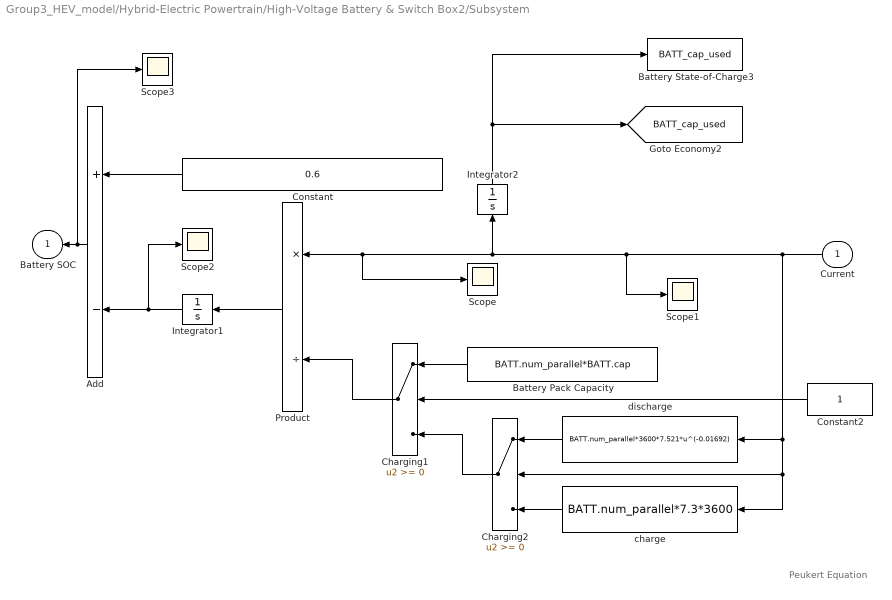
== system Group3_HEV_model/Hybrid-Electric Powertrain/High-Voltage Battery & Switch Box2/Subsystem ==
  note: Peukert Equation
  Current : Inport
  Add : Sum  Inputs=+-
  Battery Pack Capacity : Constant  Value=BATT.num_parallel*BATT.cap
  Battery State-of-Charge3 : ToWorkspace  VariableName=BATT_cap_used  SampleTime=-1
  Charging1 : Switch  SaturateOnIntegerOverflow=on  InputSameDT=on
  Charging2 : Switch  SaturateOnIntegerOverflow=on  InputSameDT=on
  Constant : Constant  Value=0.6
  Constant2 : Constant
  Integrator1 : Integrator
  Integrator2 : Integrator
  Product : Product  Inputs=*/  RndMeth=Zero
  Scope{,1..3} (4 alike) : Scope
      Scope1 settings: TimeRange=1800  YMin=-47.4434389140271  YMax=72.5565610859729  SaveName=ScopeData7
      Scope2 settings: SaveName=ScopeData8
      Scope3 settings: SaveName=ScopeData9
  charge : Fcn  Expr=BATT.num_parallel*7.3*3600
  discharge : Fcn  Expr=BATT.num_parallel*3600*7.521*u^(-0.01692)
  Battery SOC : Outport
  tag scope: BATT_cap_used=global
  wires:
  Constant/1 -> Add/1
  Product/1 -> Integrator1/1
  Add/1 -> Scope3/1, Battery SOC/1
  Current/1 -> Scope1/1, Product/1, Scope/1, Integrator2/1, discharge/1, charge/1, Charging2/2
  discharge/1 -> Charging2/1
  charge/1 -> Charging2/3
  Battery Pack Capacity/1 -> Charging1/1
  Charging1/1 -> Product/2
  Charging2/1 -> Charging1/3
  Constant2/1 -> Charging1/2
  Integrator1/1 -> Scope2/1, Add/2
  Integrator2/1 -> [BATT_cap_used], Battery State-of-Charge3/1

== system Group3_HEV_model/Hybrid-Electric Powertrain/Torque Converter/If Pump Speed > Turbine Speed (Normal Torus Flow) ==
  Pump Torque : Inport
  Turbine Speed : Inport  Port=2
  Action Port : ActionPort  ActionType=then
  Constant : Constant
  Demux : Demux  Outputs=2
  Demux1 : Demux  Outputs=2
  Fcn : Fcn  Expr=TC.thresh_T_p*(u[1])^2
  If : If  IfExpression=u1 >= 0
  Mux : Mux  Inputs=2
  Sum : Sum  Inputs=+-
  Switch1 : Switch  SaturateOnIntegerOverflow=on  InputSameDT=on
  Switch2 : Switch  SaturateOnIntegerOverflow=on  InputSameDT=on
  Torque Coupling Stage : Subsystem  TreatAsAtomicUnit=on
  Torque Multiplication Stage : Subsystem  TreatAsAtomicUnit=on
  Pump Speed : Outport  InitialOutput=0
  Turbine Torque : Outport  Port=2  InitialOutput=0
  Case : Outport  Port=3  InitialOutput=0
  wires:
  Switch2/1 -> Turbine Torque/1
  Switch1/1 -> Pump Speed/1
  Fcn/1 -> Sum/2
  Turbine Speed/1 -> Mux/2, Fcn/1
  Sum/1 -> If/1, Switch1/2, Switch2/2
  Pump Torque/1 -> Sum/1, Mux/1
  If/1 -> Torque Multiplication Stage/Action
  If/2 -> Torque Coupling Stage/Action
  Demux/2 -> Torque Multiplication Stage/2(Turbine Speed)
  Demux/1 -> Torque Multiplication Stage/1(Pump Torque)
  Demux1/1 -> Torque Coupling Stage/1(Pump Torque)
  Demux1/2 -> Torque Coupling Stage/2(Turbine Speed)
  Mux/1 -> Demux/1, Demux1/1
  Torque Coupling Stage/2(Turbine Torque) -> Switch2/3
  Torque Multiplication Stage/1(Pump Speed) -> Switch1/1
  Torque Coupling Stage/1(Pump Speed) -> Switch1/3
  Torque Multiplication Stage/2(Turbine Torque) -> Switch2/1
  Constant/1 -> Case/1

== system Group3_HEV_model/Hybrid-Electric Powertrain/Torque Converter/If Turbine Speed > Pump Speed (Reverse Torus Flow) ==
  Pump Torque : Inport
  Turbine Speed : Inport  Port=2
  Action Port : ActionPort  ActionType=elseif
  Constant : Constant  Value=2
  Fcn : Fcn  Expr=( -TC.c8*u[2] - sqrt((TC.c8*u[2])^2 - 4*TC.c9*(TC.c7*(u[2])^2 + u[1]))) / (2*TC.c9)
  Mux : Mux  Inputs=2
  Pump Speed : Outport  InitialOutput=0
  Turbine Torque : Outport  Port=2  InitialOutput=0
  Case : Outport  Port=3  InitialOutput=0
  wires:
  Mux/1 -> Fcn/1
  Fcn/1 -> Pump Speed/1
  Turbine Speed/1 -> Mux/2
  Pump Torque/1 -> Turbine Torque/1, Mux/1
  Constant/1 -> Case/1

== system Group3_HEV_model/Hybrid-Electric Powertrain/Torque Converter/Torque Converter Lock-Up ==
  Pump Torque : Inport
  Turbine Speed : Inport  Port=2
  Action Port : ActionPort  ActionType=elseif
  Constant : Constant  Value=3
  Pump Speed : Outport  InitialOutput=0
  Turbine Torque : Outport  Port=2  InitialOutput=0
  Case : Outport  Port=3  InitialOutput=0
  wires:
  Pump Torque/1 -> Turbine Torque/1
  Turbine Speed/1 -> Pump Speed/1
  Constant/1 -> Case/1

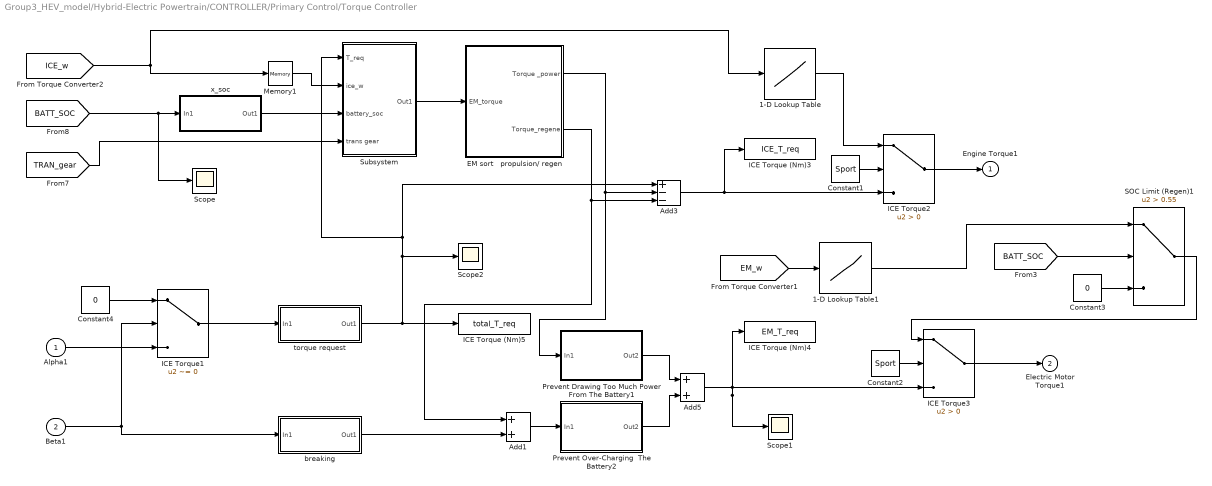
== system Group3_HEV_model/Hybrid-Electric Powertrain/CONTROLLER/Primary Control/Torque Controller ==
  Alpha1 : Inport
  Beta1 : Inport  Port=2
  1-D Lookup Table : Lookup_n-D  NumberOfTableDimensions=1  BreakpointsForDimension1=ICE.maxT_w  Table=ICE.maxT_T  RndMeth=Simplest  InputSameDT=on
  1-D Lookup Table1 : Lookup_n-D  NumberOfTableDimensions=1  BreakpointsForDimension1=EM2.maxT_w  Table=EM2.maxT_T  RndMeth=Simplest  InputSameDT=on
  Add1 : Sum
  Add3 : Sum  Inputs=+--
  Add5 : Sum
  Constant1 : Constant  Value=Sport
  Constant2 : Constant  Value=Sport
  Constant3 : Constant  Value=0
  Constant4 : Constant  Value=0
  EM sort   propulsion/ regen : Subsystem
  ICE Torque (Nm)3 : ToWorkspace  VariableName=ICE_T_req  SampleTime=-1
  ICE Torque (Nm)4 : ToWorkspace  VariableName=EM_T_req  SampleTime=-1
  ICE Torque (Nm)5 : ToWorkspace  VariableName=total_T_req  SampleTime=-1
  ICE Torque1 : Switch  Criteria=u2 ~= 0
  ICE Torque2 : Switch  Criteria=u2 > Threshold
  ICE Torque3 : Switch  Criteria=u2 > Threshold
  Memory1 : Memory
  Prevent Drawing Too Much Power From The Battery1 : Subsystem
  Prevent Over-Charging  The Battery2 : Subsystem
  SOC Limit (Regen)1 : Switch  Criteria=u2 > Threshold  Threshold=0.55
  Scope : Scope
      settings: TimeRange=4080  YMin=0.545  YMax=0.65  SaveName=ScopeData10
  Scope1 : Scope
      settings: TimeRange=4080
  Scope2 : Scope
      settings: TimeRange=4080  SaveName=ScopeData2
  Subsystem : Subsystem
  breaking : Subsystem
  torque request : Subsystem
  x_soc : Subsystem
  Engine Torque1 : Outport  InitialOutput=0
  Electric Motor Torque1 : Outport  Port=2  InitialOutput=0
  wires:
  torque request/1(Out1) -> ICE Torque (Nm)5/1, Scope2/1, Subsystem/1(T_req), Add3/1
  breaking/1(Out1) -> Add1/2
  [BATT_SOC] -> Scope/1, x_soc/1(In1)
  [ICE_w] -> Memory1/1, 1-D Lookup Table/1
  Add3/1 -> ICE Torque (Nm)3/1, ICE Torque2/3
  Subsystem/1(Out1) -> EM sort   propulsion/ regen/1(EM_torque)
  [TRAN_gear] -> Subsystem/4(trans gear)
  Memory1/1 -> Subsystem/2(ice_w)
  Prevent Drawing Too Much Power From The Battery1/1(Out2) -> Add5/1
  Beta1/1 -> breaking/1(In1), ICE Torque1/2
  Add5/1 -> ICE Torque (Nm)4/1, Scope1/1, ICE Torque3/3
  ICE Torque1/1 -> torque request/1(In1)
  Constant4/1 -> ICE Torque1/1
  Alpha1/1 -> ICE Torque1/3
  EM sort   propulsion/ regen/1(Torque _power) -> Add3/2, Prevent Drawing Too Much Power From The Battery1/1(In1)
  EM sort   propulsion/ regen/2(Torque_regene) -> Add1/1, Add3/3
  Add1/1 -> Prevent Over-Charging  The Battery2/1(In1)
  Prevent Over-Charging  The Battery2/1(Out2) -> Add5/2
  x_soc/1(Out1) -> Subsystem/3(battery_soc)
  Constant1/1 -> ICE Torque2/2
  1-D Lookup Table/1 -> ICE Torque2/1
  Constant2/1 -> ICE Torque3/2
  [EM_w] -> 1-D Lookup Table1/1
  [BATT_SOC] -> SOC Limit (Regen)1/2
  Constant3/1 -> SOC Limit (Regen)1/3
  1-D Lookup Table1/1 -> SOC Limit (Regen)1/1
  SOC Limit (Regen)1/1 -> ICE Torque3/1
  ICE Torque3/1 -> Electric Motor Torque1/1
  ICE Torque2/1 -> Engine Torque1/1

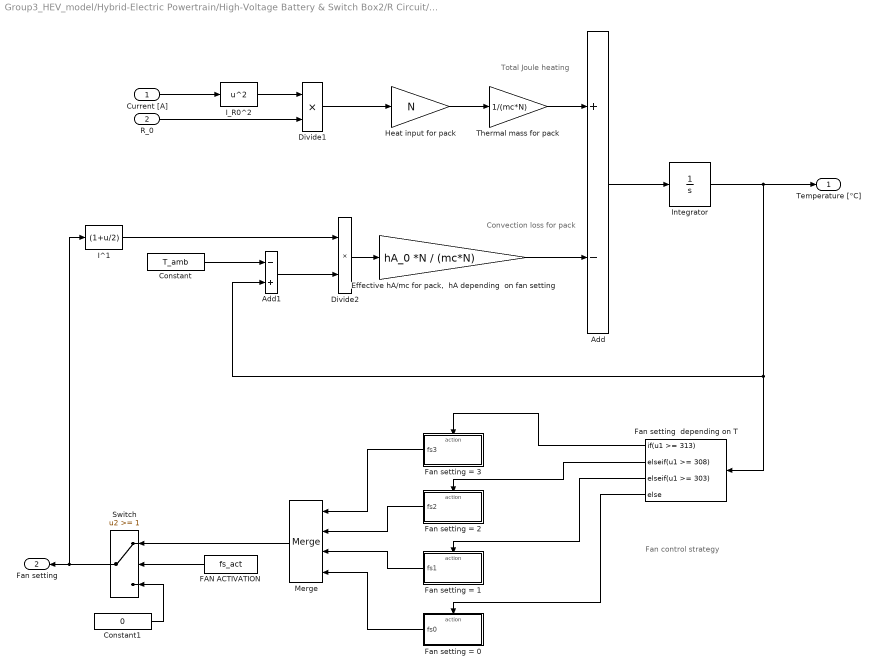
== system Group3_HEV_model/Hybrid-Electric Powertrain/High-Voltage Battery & Switch Box2/R Circuit/THERMAL MODEL ==
  note: Total Joule heating
  note: Convection loss for pack
  note: Fan control strategy
  Current [A] : Inport
  R_0 : Inport  Port=2
  Add : Sum  Inputs=+-
  Add1 : Sum  Inputs=-+
  Constant : Constant  Value=T_amb
  Constant1 : Constant  Value=0
  Divide1 : Product  Inputs=**
  Divide2 : Product  Inputs=**
  "Effective hA/mc for pack,  hA depending  on fan setting" : Gain  Gain=hA_0 *N / (mc*N)
  FAN ACTIVATION : Constant  Value=fs_act
  Fan setting  depending on T : If  IfExpression=u1 >= 313  ElseIfExpressions=u1 >= 308 , u1 >= 303
  Fan setting = 0 : Subsystem  TreatAsAtomicUnit=on
  Fan setting = 1 : Subsystem  TreatAsAtomicUnit=on
  Fan setting = 2 : Subsystem  TreatAsAtomicUnit=on
  Fan setting = 3 : Subsystem  TreatAsAtomicUnit=on
  Heat input for pack : Gain  Gain=N
  I^1 : Fcn  Expr=(1+u/2)
  I_R0^2 : Fcn  Expr=u^2
  Integrator : Integrator  InitialCondition=T_amb
  Merge : Merge  Inputs=4  InitialOutput=fs_0
  Switch : Switch  Threshold=1
  Thermal mass for pack : Gain  Gain=1/(mc*N)
  Temperature [°C] : Outport
  Fan setting : Outport  Port=2
  wires:
  Add/1 -> Integrator/1
  Integrator/1 -> Temperature [°C]/1, Fan setting  depending on T/1, Add1/2
  Current [A]/1 -> I_R0^2/1
  Thermal mass for pack/1 -> Add/1
  "Effective hA/mc for pack,  hA depending  on fan setting"/1 -> Add/2
  Constant/1 -> Add1/1
  R_0/1 -> Divide1/2
  Divide1/1 -> Heat input for pack/1
  I_R0^2/1 -> Divide1/1
  Heat input for pack/1 -> Thermal mass for pack/1
  Fan setting  depending on T/1 -> Fan setting = 3/Action
  Fan setting  depending on T/2 -> Fan setting = 2/Action
  Fan setting  depending on T/3 -> Fan setting = 1/Action
  Fan setting  depending on T/4 -> Fan setting = 0/Action
  Fan setting = 3/1(fs3) -> Merge/1
  Fan setting = 2/1(fs2) -> Merge/2
  Fan setting = 1/1(fs1) -> Merge/3
  Fan setting = 0/1(fs0) -> Merge/4
  Merge/1 -> Switch/1
  Switch/1 -> Fan setting/1, I^1/1
  Constant1/1 -> Switch/3
  FAN ACTIVATION/1 -> Switch/2
  Divide2/1 -> "Effective hA/mc for pack,  hA depending  on fan setting"/1
  Add1/1 -> Divide2/2
  I^1/1 -> Divide2/1

== system Group3_HEV_model/Hybrid-Electric Powertrain/Torque Converter/If Pump Speed > Turbine Speed (Normal Torus Flow)/Torque Coupling Stage ==
  Pump Torque : Inport
  Turbine Speed : Inport  Port=2
  Action Port : ActionPort  ActionType=else
  Fcn1 : Fcn  Expr=( -TC.c8*u[2] + sqrt((TC.c8*u[2])^2 - 4*TC.c7*(TC.c9*(u[2])^2 - u[1]))) / (2*TC.c7)
  Mux : Mux  Inputs=2
  Pump Speed : Outport  InitialOutput=0
  Turbine Torque : Outport  Port=2  InitialOutput=0
  wires:
  Pump Torque/1 -> Mux/1, Turbine Torque/1
  Turbine Speed/1 -> Mux/2
  Mux/1 -> Fcn1/1
  Fcn1/1 -> Pump Speed/1

== system Group3_HEV_model/Hybrid-Electric Powertrain/Torque Converter/If Pump Speed > Turbine Speed (Normal Torus Flow)/Torque Multiplication Stage ==
  Pump Torque : Inport
  Turbine Speed : Inport  Port=2
  Action Port : ActionPort  ActionType=then
  Fcn : Fcn  Expr=( -TC.c5*u[2] + sqrt((TC.c5*u[2])^2 - 4*TC.c4*(TC.c6*(u[2])^2 - u[1]))) / (2*TC.c4)
  Fcn1 : Fcn  Expr=TC.c1*(u[1])^2 + TC.c2*u[1]*u[2] + TC.c3*(u[2])^2
  Mux : Mux  Inputs=2
  Mux1 : Mux  Inputs=2
  Pump Speed : Outport  InitialOutput=0
  Turbine Torque : Outport  Port=2  InitialOutput=0
  wires:
  Fcn/1 -> Pump Speed/1, Mux1/1
  Pump Torque/1 -> Mux/1
  Turbine Speed/1 -> Mux/2, Mux1/2
  Mux/1 -> Fcn/1
  Fcn1/1 -> Turbine Torque/1
  Mux1/1 -> Fcn1/1
